simulink model "ModelanfisNDEF"  (R2017a)
settings: Solver=VariableStepAuto  StartTime=0.0  StopTime=577  RelTol=1e-3
values from neighbouring files (symbols this model uses):
  dinnegc12 = [-0.01 -0.01 -0.02 -0.01 -0.01 -0.01 0 0 0 0 0.01 -0.01 ... (2312 elements, 578x4)]    [anfisd.mat]    (also in anfisfin.mat; cinco.mat)
libraries: dspsrcs4 x36, fuzblock x12
settings Model: Creator=Dell  LastModifiedBy=Dell

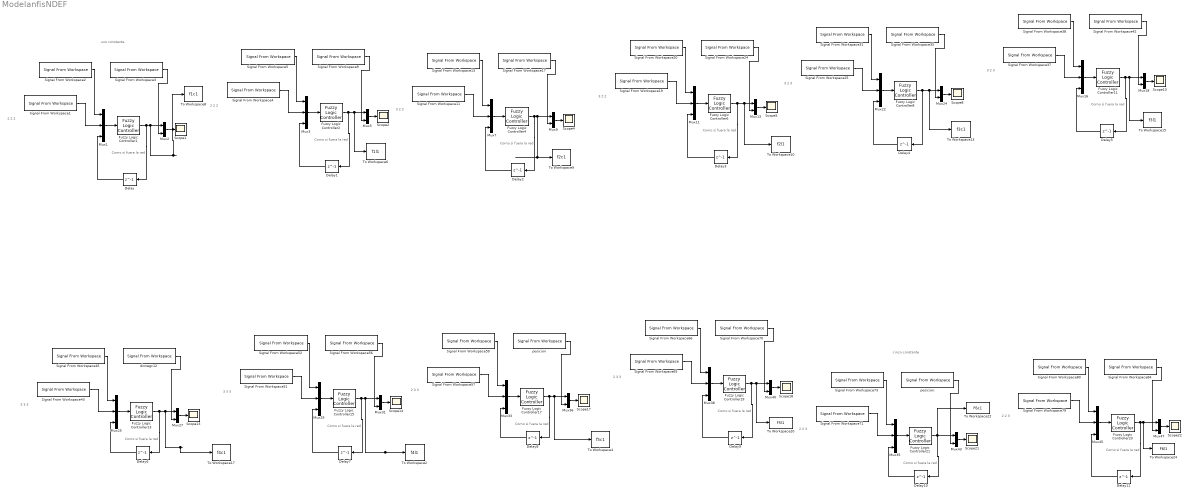
== system ModelanfisNDEF ==
  note: uno constante
  note: 2 2 2
  note: Como si fuera la red
  note: 2 2 2
  note: Como si fuera la red
  note: 3 2 2
  note: Como si fuera la red
  note: 3 2 2
  note: Como si fuera la red
  note: 3 2 3
  note: 3 2 3
  note: Como si fuera la red
  note: 3 3 3
  note: Como si fuera la red
  note: 3 3 3
  note: Como si fuera la red
  note: 2 3 3
  note: Como si fuera la red
  note: 2 3 3
  note: Como si fuera la red
  note: cinco constante
  note: 2 2 3
  note: Como si fuera la red
  note: 2 2 3
  note: Como si fuera la red
  Delay{,1..11} (12 alike) : Delay  DelayLength=1  InitialCondition=0
  Fuzzy Logic Controller1 : fuzblock/Fuzzy Logic  Controller  fis=Uno1
  Fuzzy Logic Controller11 : fuzblock/Fuzzy Logic  Controller  fis=tres3
  Fuzzy Logic Controller13 : fuzblock/Fuzzy Logic  Controller  fis=cuatro
  Fuzzy Logic Controller15 : fuzblock/Fuzzy Logic  Controller  fis=cuatro4
  Fuzzy Logic Controller17 : fuzblock/Fuzzy Logic  Controller  fis=cinco
  Fuzzy Logic Controller19 : fuzblock/Fuzzy Logic  Controller  fis=cinco5
  Fuzzy Logic Controller2 : fuzblock/Fuzzy Logic  Controller  fis=Uno1
  Fuzzy Logic Controller21 : fuzblock/Fuzzy Logic  Controller  fis=seis
  Fuzzy Logic Controller23 : fuzblock/Fuzzy Logic  Controller  fis=seis6
  Fuzzy Logic Controller4 : fuzblock/Fuzzy Logic  Controller  fis=dos2
  Fuzzy Logic Controller6 : fuzblock/Fuzzy Logic  Controller  fis=dos2
  Fuzzy Logic Controller8 : fuzblock/Fuzzy Logic  Controller  fis=tres
  Mux{1,3,7,11,16,22,25,29,33,35,38,45} (12 alike) : Mux  Inputs=3
  Mux{2,5,9,13,18,24,27,31,36,40,43,47} (12 alike) : Mux  Inputs=2
  Scope{1..2,4..5,8,10,13..14,17..18,21..22} (12 alike) : Scope
  Signal From Workspace{1,4,11,19,25,37,43,51,57,65,71,79} (12 alike) : dspsrcs4/Signal From Workspace  X=dinnegc12(:,2)  Ts=1  nsamps=1  OutputAfterFinalValue=Setting to zero  ignoreOrWarnInputAndFrameLengths=off  OutputFrames=off
  Signal From Workspace{2,5,13,20,31,38,45,52,59,66,73,80} (12 alike) : dspsrcs4/Signal From Workspace  X=dinnegc12(:,1)  Ts=1  nsamps=1  OutputAfterFinalValue=Setting to zero  ignoreOrWarnInputAndFrameLengths=off  OutputFrames=off
  Signal From Workspace{3,9,17,24,35,42,56,70,84} (9 alike) : dspsrcs4/Signal From Workspace  X=dinnegc12(:,4)  Ts=1  nsamps=1  OutputAfterFinalValue=Setting to zero  ignoreOrWarnInputAndFrameLengths=off  OutputFrames=off
  To Workspace10 : ToWorkspace  VariableName=f2l1  SampleTime=-1
      settings: Save2DSignal=2-D array (concatenate along first dimension)
  To Workspace13 : ToWorkspace  VariableName=f3c1  SampleTime=-1
      settings: Save2DSignal=2-D array (concatenate along first dimension)
  To Workspace15 : ToWorkspace  VariableName=f3l1  SampleTime=-1
      settings: Save2DSignal=2-D array (concatenate along first dimension)
  To Workspace17 : ToWorkspace  VariableName=f4c1  SampleTime=-1
      settings: Save2DSignal=2-D array (concatenate along first dimension)
  To Workspace2 : ToWorkspace  VariableName=f4l1  SampleTime=-1
      settings: Save2DSignal=2-D array (concatenate along first dimension)
  To Workspace20 : ToWorkspace  VariableName=F5l1  SampleTime=-1
  To Workspace22 : ToWorkspace  VariableName=F6c1  SampleTime=-1
  To Workspace24 : ToWorkspace  VariableName=F6l1  SampleTime=-1
  To Workspace4 : ToWorkspace  VariableName=f5c1  SampleTime=-1
      settings: Save2DSignal=2-D array (concatenate along first dimension)
  To Workspace6 : ToWorkspace  VariableName=f1l1  SampleTime=-1
      settings: Save2DSignal=2-D array (concatenate along first dimension)
  To Workspace8 : ToWorkspace  VariableName=f1c1  SampleTime=-1
      settings: Save2DSignal=2-D array (concatenate along first dimension)
  To Workspace9 : ToWorkspace  VariableName=f2c1  SampleTime=-1
      settings: Save2DSignal=2-D array (concatenate along first dimension)
  dinnegc12 : dspsrcs4/Signal From Workspace  X=dinnegc12(:,4)  Ts=1  nsamps=1  OutputAfterFinalValue=Setting to zero  ignoreOrWarnInputAndFrameLengths=off  OutputFrames=off
  "posicion " : dspsrcs4/Signal From Workspace  X=dinnegc12(:,4)  Ts=1  nsamps=1  OutputAfterFinalValue=Setting to zero  ignoreOrWarnInputAndFrameLengths=off  OutputFrames=off
  posicion. : dspsrcs4/Signal From Workspace  X=dinnegc12(:,4)  Ts=1  nsamps=1  OutputAfterFinalValue=Setting to zero  ignoreOrWarnInputAndFrameLengths=off  OutputFrames=off
  wires:
  Mux1/1 -> Fuzzy Logic Controller1/1
  Signal From Workspace3/1 -> Mux2/2
  Mux2/1 -> Scope1/1
  Signal From Workspace2/1 -> Mux1/1
  Fuzzy Logic Controller1/1 -> Delay/1, To Workspace8/1, Mux2/1
  Signal From Workspace1/1 -> Mux1/2
  Delay/1 -> Mux1/3
  Delay1/1 -> Mux3/3
  Signal From Workspace4/1 -> Mux3/2
  Fuzzy Logic Controller2/1 -> To Workspace6/1, Mux5/1, Delay1/1
  Signal From Workspace5/1 -> Mux3/1
  Mux5/1 -> Scope2/1
  Signal From Workspace9/1 -> Mux5/2
  Mux3/1 -> Fuzzy Logic Controller2/1
  Mux11/1 -> Fuzzy Logic Controller6/1
  Signal From Workspace24/1 -> Mux13/2
  Mux13/1 -> Scope5/1
  Signal From Workspace20/1 -> Mux11/1
  Fuzzy Logic Controller6/1 -> Delay3/1, To Workspace10/1, Mux13/1
  Signal From Workspace19/1 -> Mux11/2
  Delay3/1 -> Mux11/3
  Delay2/1 -> Mux7/3
  Signal From Workspace11/1 -> Mux7/2
  Fuzzy Logic Controller4/1 -> To Workspace9/1, Mux9/1, Delay2/1
  Signal From Workspace13/1 -> Mux7/1
  Mux9/1 -> Scope4/1
  Signal From Workspace17/1 -> Mux9/2
  Mux7/1 -> Fuzzy Logic Controller4/1
  Mux22/1 -> Fuzzy Logic Controller8/1
  Signal From Workspace35/1 -> Mux24/2
  Mux24/1 -> Scope8/1
  Signal From Workspace31/1 -> Mux22/1
  Fuzzy Logic Controller8/1 -> Delay4/1, To Workspace13/1, Mux24/1
  Signal From Workspace25/1 -> Mux22/2
  Delay4/1 -> Mux22/3
  Delay5/1 -> Mux16/3
  Signal From Workspace37/1 -> Mux16/2
  Fuzzy Logic Controller11/1 -> Delay5/1, To Workspace15/1, Mux18/1
  Signal From Workspace38/1 -> Mux16/1
  Mux18/1 -> Scope10/1
  Signal From Workspace42/1 -> Mux18/2
  Mux16/1 -> Fuzzy Logic Controller11/1
  Mux29/1 -> Fuzzy Logic Controller15/1
  Signal From Workspace56/1 -> Mux31/2
  Mux31/1 -> Scope14/1
  Signal From Workspace52/1 -> Mux29/1
  Fuzzy Logic Controller15/1 -> Delay7/1, To Workspace2/1, Mux31/1
  Signal From Workspace51/1 -> Mux29/2
  Delay7/1 -> Mux29/3
  Delay6/1 -> Mux25/3
  Signal From Workspace43/1 -> Mux25/2
  Fuzzy Logic Controller13/1 -> To Workspace17/1, Mux27/1, Delay6/1
  Signal From Workspace45/1 -> Mux25/1
  Mux27/1 -> Scope13/1
  dinnegc12/1 -> Mux27/2
  Mux25/1 -> Fuzzy Logic Controller13/1
  Mux33/1 -> Fuzzy Logic Controller17/1
  "posicion "/1 -> Mux36/2
  Mux36/1 -> Scope17/1
  Signal From Workspace59/1 -> Mux33/1
  Signal From Workspace57/1 -> Mux33/2
  Delay8/1 -> Mux33/3
  Delay9/1 -> Mux38/3
  Signal From Workspace65/1 -> Mux38/2
  Fuzzy Logic Controller19/1 -> To Workspace20/1, Mux40/1, Delay9/1
  Signal From Workspace66/1 -> Mux38/1
  Mux40/1 -> Scope18/1
  Signal From Workspace70/1 -> Mux40/2
  Mux38/1 -> Fuzzy Logic Controller19/1
  Mux45/1 -> Fuzzy Logic Controller23/1
  Signal From Workspace84/1 -> Mux47/2
  Mux47/1 -> Scope22/1
  Signal From Workspace80/1 -> Mux45/1
  Fuzzy Logic Controller23/1 -> Delay11/1, To Workspace24/1, Mux47/1
  Signal From Workspace79/1 -> Mux45/2
  Delay11/1 -> Mux45/3
  Delay10/1 -> Mux35/3
  Signal From Workspace71/1 -> Mux35/2
  Fuzzy Logic Controller21/1 -> To Workspace22/1, Mux43/1, Delay10/1
  Signal From Workspace73/1 -> Mux35/1
  Mux43/1 -> Scope21/1
  posicion./1 -> Mux43/2
  Mux35/1 -> Fuzzy Logic Controller21/1
  Fuzzy Logic Controller17/1 -> Delay8/1, To Workspace4/1, Mux36/1
